simulink model "gyroboy"  (R2019a)
settings: Solver=ode45  StartTime=0.0  StopTime=10.0  RelTol=1e-3
PreLoadFcn:
  | config
  | preload
InitFcn:
  | plant
  | control
values from neighbouring files (symbols this model uses):
  K = lqr(s4, QQ, RR)    [control.m]
undefined symbols (not defined in the file or in its folder): A1, A2, B1, B2, C1, C2, D1, D2, K_PWM, Psi0, R, W
libraries: simulink_extras x2
settings Model: Creator=roslovetspv  LastModifiedBy=Pavel Roslovets
settings SolverCC: ZeroCrossAlgorithm=Adaptive
settings DataIOCC: ReturnWorkspaceOutputs=off
settings DebuggingCC: ArithmeticOperatorsInVariantConditions=warning
settings SFSimCC: SimUseLocalCustomCode=off
settings RTWCC: RTWUseLocalCustomCode=off
settings CodeAppCC: StateflowObjectComments=on

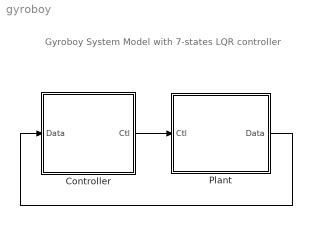
== system gyroboy ==
  note: Gyroboy System Model
      | with 7-states LQR controller
  Controller : Subsystem
  Plant : Subsystem
  wires:
  Controller/1(Ctl) -> Plant/1(Ctl)
  Plant/1(Data) -> Controller/1(Data)

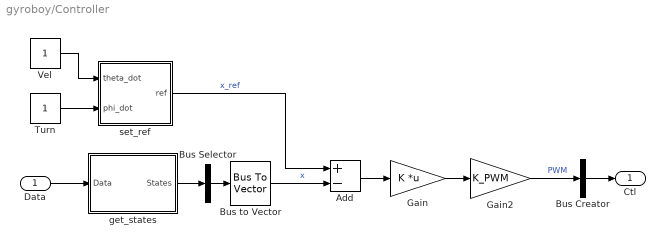
== system gyroboy/Controller ==
  Data : Inport
  Add : Sum  Inputs=+-
  Bus Creator : BusCreator  Inputs=1  OutDataTypeStr=Bus: Ctl
      settings: InheritFromInputs=off
  Bus Selector : BusSelector  OutputSignals=theta_int,theta,psi,theta_dot,psi_dot,phi,phi_dot  OutputAsBus=on
  Bus to Vector : BusToVector
  Gain : Gain  Gain=K  Multiplication=Matrix(K*u)
  Gain2 : Gain  Gain=K_PWM
  Turn : Constant
  Vel : Constant
  get_states : Subsystem
  set_ref : Subsystem
  Ctl : Outport
  wires:
  Bus Creator/1 -> Ctl/1
  Data/1 -> get_states/1(Data)
  get_states/1(States) -> Bus Selector/1
  Add/1 -> Gain/1
  Bus to Vector/1 -> Add/2  "x"
  Bus Selector/1 -> Bus to Vector/1
  Gain/1 -> Gain2/1
  Gain2/1 -> Bus Creator/1  "PWM"
  Vel/1 -> set_ref/1(theta_dot)
  Turn/1 -> set_ref/2(phi_dot)
  set_ref/1(ref) -> Add/1  "x_ref"

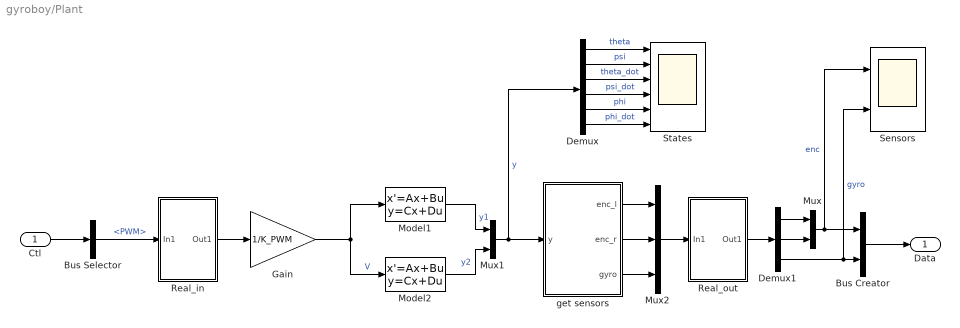
== system gyroboy/Plant ==
  Ctl : Inport
  Bus Creator : BusCreator  Inputs=2
  Bus Selector : BusSelector  OutputSignals=PWM
  Demux : Demux  Outputs=6
  Demux1 : Demux  Outputs=3
  Gain : Gain  Gain=1/K_PWM
  Model1 : StateSpace  A=A1  B=B1  C=C1  D=D1  InitialCondition=[0 Psi0 0 0]
  Model2 : StateSpace  A=A2  B=B2  C=C2  D=D2  InitialCondition=0
  Mux : Mux  Inputs=2
  Mux1 : Mux  Inputs=2
  Mux2 : Mux  Inputs=3
  Real_in : Subsystem  Variant=on  VariantControl=Variant1
  Real_out : Subsystem  Variant=on  VariantControl=Variant1
  Sensors : Scope  NumInputPorts=2
  States : Scope  NumInputPorts=6
  get sensors : MATLAB Function  TreatAsAtomicUnit=on
  Data : Outport
  wires:
  Model1/1 -> Mux1/1  "y1"
  Model2/1 -> Mux1/2  "y2"
  Gain/1 -> Model2/1, Model1/1  "V"
  Real_in/1(" Out1") -> Gain/1
  Ctl/1 -> Bus Selector/1
  Mux1/1 -> Demux/1, get sensors/1(y)  "y"
  Mux2/1 -> Real_out/1("In1 ")
  get sensors/3(gyro) -> Mux2/3
  Real_out/1(" Out1") -> Demux1/1
  Demux/4 -> States/4  "psi_dot"
  Demux/6 -> States/6  "phi_dot"
  Demux/5 -> States/5  "phi"
  Bus Creator/1 -> Data/1
  Demux1/1 -> Mux/1
  Demux1/2 -> Mux/2
  Demux1/3 -> Sensors/2, Bus Creator/2  "gyro"
  Demux/2 -> States/2  "psi"
  Demux/3 -> States/3  "theta_dot"
  Demux/1 -> States/1  "theta"
  Bus Selector/1 -> Real_in/1("In1 ")  "<PWM>"
  get sensors/1(enc_l) -> Mux2/1
  get sensors/2(enc_r) -> Mux2/2
  Mux/1 -> Sensors/1, Bus Creator/1  "enc"

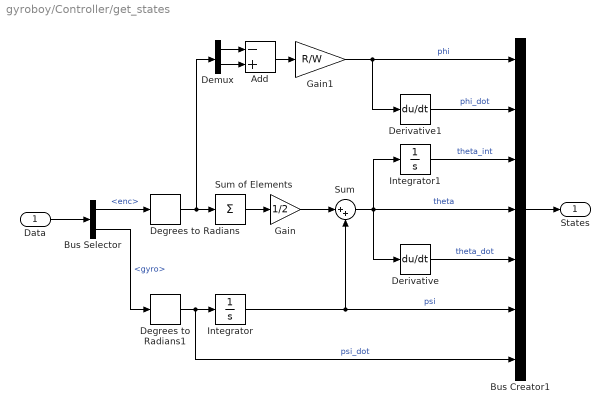
== system gyroboy/Controller/get_states ==
  Data : Inport
  Add : Sum  Inputs=-+
  Bus Creator1 : BusCreator  Inputs=7
  Bus Selector : BusSelector  OutputSignals=enc,gyro
  Degrees to Radians : simulink_extras/Transformations/Degrees to Radians
  Degrees to Radians1 : simulink_extras/Transformations/Degrees to Radians
  Demux : Demux  Outputs=2
  Derivative : Derivative
  Derivative1 : Derivative
  Gain : Gain  Gain=1/2
  Gain1 : Gain  Gain=R/W
  Integrator : Integrator
  Integrator1 : Integrator
  Sum : Sum  Inputs=|++
  Sum of Elements : Sum  Inputs=+
  States : Outport
  wires:
  Gain/1 -> Sum/1
  Degrees to Radians/1 -> Demux/1, Sum of Elements/1
  Integrator/1 -> Sum/2, Bus Creator1/6  "psi"
  Data/1 -> Bus Selector/1
  Bus Selector/1 -> Degrees to Radians/1  "<enc>"
  Sum/1 -> Integrator1/1, Derivative/1, Bus Creator1/4  "theta"
  Derivative/1 -> Bus Creator1/5  "theta_dot"
  Bus Creator1/1 -> States/1
  Sum of Elements/1 -> Gain/1
  Degrees to Radians1/1 -> Bus Creator1/7, Integrator/1  "psi_dot"
  Bus Selector/2 -> Degrees to Radians1/1  "<gyro>"
  Integrator1/1 -> Bus Creator1/3  "theta_int"
  Demux/1 -> Add/1
  Demux/2 -> Add/2
  Add/1 -> Gain1/1
  Gain1/1 -> Derivative1/1, Bus Creator1/1  "phi"
  Derivative1/1 -> Bus Creator1/2  "phi_dot"

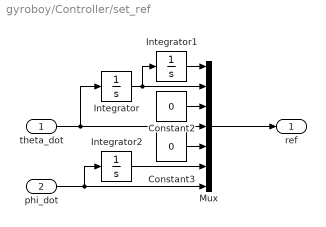
== system gyroboy/Controller/set_ref ==
  theta_dot : Inport
  phi_dot : Inport  Port=2
  Constant2 : Constant  Value=0
  Constant3 : Constant  Value=0
  Integrator : Integrator
  Integrator1 : Integrator
  Integrator2 : Integrator
  Mux : Mux  Inputs=7
  ref : Outport
  wires:
  Constant2/1 -> Mux/3
  Constant3/1 -> Mux/5
  Mux/1 -> ref/1
  Integrator/1 -> Integrator1/1, Mux/2
  phi_dot/1 -> Integrator2/1, Mux/7
  Integrator2/1 -> Mux/6
  Integrator1/1 -> Mux/1
  theta_dot/1 -> Integrator/1, Mux/4

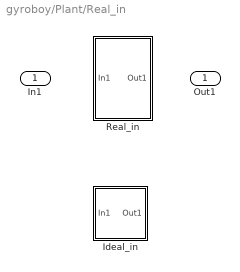
== system gyroboy/Plant/Real_in ==
  "In1 " : Inport
  Ideal_in : Subsystem  VariantControl=(default)
  Real_in : Subsystem  VariantControl=real_model == 1
  " Out1" : Outport

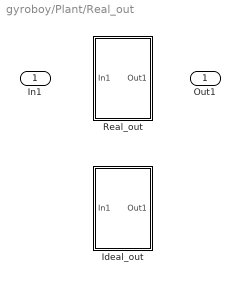
== system gyroboy/Plant/Real_out ==
  "In1 " : Inport
  Ideal_out : Subsystem  VariantControl=(default)
  Real_out : Subsystem  VariantControl=real_model == 1
  " Out1" : Outport

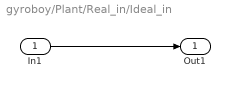
== system gyroboy/Plant/Real_in/Ideal_in ==
  "In1 " : Inport
  " Out1" : Outport
  wires:
  "In1 "/1 -> " Out1"/1

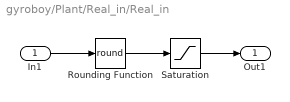
== system gyroboy/Plant/Real_in/Real_in ==
  In1 : Inport
  Rounding Function : Rounding  Operator=round
  Saturation : Saturate  UpperLimit=100  LowerLimit=-100
  Out1 : Outport
  wires:
  In1/1 -> Rounding Function/1
  Saturation/1 -> Out1/1
  Rounding Function/1 -> Saturation/1

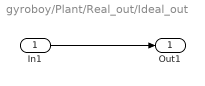
== system gyroboy/Plant/Real_out/Ideal_out ==
  In1 : Inport
  Out1 : Outport
  wires:
  In1/1 -> Out1/1

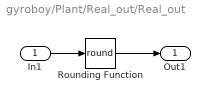
== system gyroboy/Plant/Real_out/Real_out ==
  In1 : Inport
  Rounding Function : Rounding  Operator=round
  Out1 : Outport
  wires:
  In1/1 -> Rounding Function/1
  Rounding Function/1 -> Out1/1

== matlab function gyroboy/Plant/get sensors ==
  data: enc_l output; enc_r output; y input; gyro output; R parameter; W parameter
function [enc_l, enc_r, gyro] = sensors(y, R, W)
enc_l = rad2deg(y(1) - W/R/2 * y(5) - y(2));
enc_r = rad2deg(y(1) + W/R/2 * y(5) - y(2));
gyro  = rad2deg(y(4));
